simulink model "TorqueVect_HIL_CAN"  (R2022a)
settings: Solver=VariableStepAuto  StartTime=0.0  StopTime=300  RelTol=1e-3
PreLoadFcn:
  | run('Parameters\FSE_Parameters.m')
values from neighbouring files (symbols this model uses):
  Kd = 0;')    [open_carmaker_gui.m]
  Ki = 0    [open_carmaker_gui.m]
undefined symbols (not defined in the file or in its folder): BRegenEnabledButton, canChannel, CyalphaLookUp, efficiency, Fz_curve, Fz_scaling_long, gearR, izz, jw, kd, ki, Kp, kp, l_f, l_r, lambda, m, Mz_max, N, N_lat, N_long, P_max, pid_kd_lat, pid_kd_long, pid_ki_lat, pid_ki_long, pid_kp_lat, pid_kp_long, R_max, rw, steerR, T_i_max, TC_Decr_Gas, TC_Derivative, TC_Incr_Gas, TC_On, TC_Relay_Off, TC_Relay_On, tireCornerStiffness, Ts, TV_On, TV_Override, velocity_lookup, velocity_lookup_lat, y_ref, yrr_scaling
libraries: simulink x218, slpidlib x135, CarMaker4SL x73, TractionControlLibrary x13, canmsglib x11, canlib x10, TorqueVectoringLibrary x6, simulink_extras x4, PedalConversionLibrary x3, PowerControlLibrary x1
(part 19 of 26)

== system TorqueVect_HIL_CAN/CarMaker/IPG Vehicle/PowerTrain/PTControl Example/PTControl_PC_MFE/Subsystem/PowerControl/RegenError ==
  PTotal : Inport  Unit=W  PortDimensions=1
      settings: AttributesFormatString=%<Unit>
  FF_RC : Inport  Port=2
  PRegenLimit : Inport  Port=3  OutMin=0  OutMax=80000  Unit=W  PortDimensions=1
      settings: AttributesFormatString=[%<OutMin>, %<OutMax>] %<Unit>
  rThrottle : Inport  Port=4
  Product : Product
  Product6 : Product
  Saturation : Saturate  UpperLimit=0  LowerLimit=-250000
  Saturation7 : Saturate  UpperLimit=0  LowerLimit=-250000
      settings: AttributesFormatString=[%<LowerLimit>, %<UpperLimit>] W
  Subtract1 : Sum  Inputs=+-
  PRegenError : Outport  Unit=W  PortDimensions=1
      settings: AttributesFormatString=%<Unit>
  wires:
  Saturation/1 -> Subtract1/2
  PRegenLimit/1 -> Product/2
  rThrottle/1 -> Product/1
  Product/1 -> Saturation/1
  Subtract1/1 -> Saturation7/1
  PTotal/1 -> Product6/1
  Product6/1 -> Subtract1/1
  FF_RC/1 -> Product6/2
  Saturation7/1 -> PRegenError/1  "regen error"

== system TorqueVect_HIL_CAN/CarMaker/IPG Vehicle/PowerTrain/PTControl Example/PTControl_PC_MFE/Subsystem/PowerControl/ResetPID_PC ==
  rThrottlePedal : Inport
  BRegenEnabled : Inport  Port=2
  Derivative : Derivative
  Derivative1 : Derivative
  Detect Fall Negative : simulink/Logic and Bit Operations/Detect Fall Negative  vinit=0  OutDataTypeStr=boolean
      settings: SourceProductBaseCode=SL
  Detect Fall Negative1 : simulink/Logic and Bit Operations/Detect Fall Negative  vinit=0  OutDataTypeStr=boolean
      settings: SourceProductBaseCode=SL
  OR : Logic  Operator=OR  IconShape=distinctive  AllPortsSameDT=off  OutDataTypeStr=boolean
  ResetPID_PC : Outport
  wires:
  BRegenEnabled/1 -> Derivative/1
  Detect Fall Negative/1 -> OR/1  "regen_enable_or"
  Derivative1/1 -> Detect Fall Negative1/1
  rThrottlePedal/1 -> Derivative1/1
  Derivative/1 -> Detect Fall Negative/1
  Detect Fall Negative1/1 -> OR/2  "accel_pedal_falling_or"
  OR/1 -> ResetPID_PC/1

== system TorqueVect_HIL_CAN/CarMaker/IPG Vehicle/PowerTrain/PTControl Example/PTControl_PC_MFE/Subsystem/PowerControl/TotalPower ==
  MMotorFL : Inport  OutMin=-42  OutMax=42  Unit=N*m  PortDimensions=1
      settings: AttributesFormatString=[%<OutMin>, %<OutMax>] %<Unit>
  nMotorFL : Inport  Port=2  OutMin=-3000  OutMax=3000  Unit=rad/s  PortDimensions=1
      settings: AttributesFormatString=[%<OutMin>, %<OutMax>] %<Unit>
  MMotorFR : Inport  Port=3  OutMin=-42  OutMax=42  Unit=N*m  PortDimensions=1
      settings: AttributesFormatString=[%<OutMin>, %<OutMax>] %<Unit>
  nMotorFR : Inport  Port=4  OutMin=-3000  OutMax=3000  Unit=rad/s  PortDimensions=1
      settings: AttributesFormatString=[%<OutMin>, %<OutMax>] %<Unit>
  MMotorRL : Inport  Port=5  OutMin=-42  OutMax=42  Unit=N*m  PortDimensions=1
      settings: AttributesFormatString=[%<OutMin>, %<OutMax>] %<Unit>
  nMotorRL : Inport  Port=6  OutMin=-3000  OutMax=3000  Unit=rad/s  PortDimensions=1
      settings: AttributesFormatString=[%<OutMin>, %<OutMax>] %<Unit>
  MMotorRR : Inport  Port=7  OutMin=-42  OutMax=42  Unit=N*m  PortDimensions=1
      settings: AttributesFormatString=[%<OutMin>, %<OutMax>] %<Unit>
  nMotorRR : Inport  Port=8  OutMin=-3000  OutMax=3000  Unit=rad/s  PortDimensions=1
      settings: AttributesFormatString=[%<OutMin>, %<OutMax>] %<Unit>
  PMeasured : Inport  Port=9  OutMin=-250000  OutMax=250000  Unit=W  PortDimensions=1
      settings: AttributesFormatString=[%<OutMin>, %<OutMax>] %<Unit>
  BMeasuredEnable : Inport  Port=10  OutMin=0  OutMax=1  PortDimensions=1
      settings: AttributesFormatString=[%<OutMin> / %<OutMax>]
  Product{2,7..9} (4 alike) : Product
  Saturation{1,3..5} (4 alike) : Saturate  UpperLimit=250000  LowerLimit=0
  Sum1 : Sum  Inputs=++++
  Sum3 : Sum  Inputs=++++
  Switch : Switch  Threshold=1  SaturateOnIntegerOverflow=off  InputSameDT=off
  Switch3 : Switch  Threshold=1  SaturateOnIntegerOverflow=off  InputSameDT=off
  PPositiveTotal : Outport  OutMin=0  OutMax=250000  Unit=W  PortDimensions=1
      settings: AttributesFormatString=[%<OutMin>, %<OutMax>] %<Unit>
  PTotal : Outport  Port=2  OutMin=-250000  OutMax=250000  Unit=W  PortDimensions=1
      settings: AttributesFormatString=[%<OutMin>, %<OutMax>] %<Unit>
  wires:
  MMotorRR/1 -> Product9/2
  nMotorRR/1 -> Product9/1
  nMotorRL/1 -> Product8/2
  MMotorRL/1 -> Product8/1
  nMotorFR/1 -> Product7/2
  MMotorFR/1 -> Product7/1
  nMotorFL/1 -> Product2/2
  MMotorFL/1 -> Product2/1
  Product9/1 -> Saturation5/1, Sum1/4
  Product8/1 -> Saturation4/1, Sum1/3
  Product7/1 -> Saturation3/1, Sum1/2
  BMeasuredEnable/1 -> Switch/2, Switch3/2
  Switch3/1 -> PTotal/1
  PMeasured/1 -> Switch/1, Switch3/1
  Switch/1 -> PPositiveTotal/1
  Sum1/1 -> Switch3/3  "tot_powerrrr_RC"
  Saturation1/1 -> Sum3/1
  Saturation4/1 -> Sum3/3
  Product2/1 -> Saturation1/1, Sum1/1
  Saturation5/1 -> Sum3/4
  Sum3/1 -> Switch/3  "tot_powerrrr_PC"
  Saturation3/1 -> Sum3/2

== system TorqueVect_HIL_CAN/CarMaker/IPG Vehicle/PowerTrain/PTControl Example/PTControl_PC_MFE/Subsystem/PowerControl/WheelTorqueOut ==
  PReductionF : Inport
  PReductionR : Inport  Port=2
  nMotorFL : Inport  Port=3
  nMotorFR : Inport  Port=4
  nMotorRL : Inport  Port=5
  nMotorRR : Inport  Port=6
  Divide{1..4} (4 alike) : Product  Inputs=*/
  Gain : Gain  Gain=0.5
  Gain1 : Gain  Gain=0.5
  Saturation{1..4} (4 alike) : Saturate  UpperLimit=30000  LowerLimit=1
  MReductionMotorFL : Outport
  MReductionMotorFR : Outport  Port=2
  MReductionMotorRL : Outport  Port=3
  MReductionMotorRR : Outport  Port=4
  wires:
  Divide4/1 -> MReductionMotorRR/1
  Divide3/1 -> MReductionMotorRL/1
  Divide2/1 -> MReductionMotorFR/1
  Divide1/1 -> MReductionMotorFL/1
  Saturation4/1 -> Divide4/2
  Saturation3/1 -> Divide3/2
  nMotorRR/1 -> Saturation4/1
  nMotorRL/1 -> Saturation3/1
  Gain1/1 -> Divide3/1, Divide4/1
  Saturation2/1 -> Divide2/2
  Saturation1/1 -> Divide1/2
  nMotorFR/1 -> Saturation2/1
  nMotorFL/1 -> Saturation1/1
  Gain/1 -> Divide1/1, Divide2/1
  PReductionR/1 -> Gain1/1
  PReductionF/1 -> Gain/1

== system TorqueVect_HIL_CAN/CarMaker/IPG Vehicle/PowerTrain/PTControl Example/PTControl_PC_TC_MFE/New TC/TC R1/traction_controller ==
  max_torque : Inport
  dslip : Inport  Port=2
  enable_tc : Inport  Port=3
  Kp : Inport  Port=4
  Kd : Inport  Port=5
  Add : Sum  Inputs=+-
  Saturation Dynamic : simulink/Discontinuities/Saturation Dynamic  OutMin=[]  OutMax=[]  OutDataTypeStr=Inherit: Same as second input  OutDataType=fixdt(1, 16)  OutScaling=2^-10  DoSatur=off
  min_torque : Constant  Value=0
  traction_controller : Subsystem  TreatAsAtomicUnit=on
  delta_torque : Outport  VectorParamsAs1DForOutWhenUnconnected=off
  wires:
  Kd/1 -> traction_controller/4(Kd)
  enable_tc/1 -> traction_controller/2(enable_tc)
  Kp/1 -> traction_controller/3(Kp)
  traction_controller/1(delta_torque) -> Add/2
  dslip/1 -> traction_controller/1(dslip)
  Saturation Dynamic/1 -> delta_torque/1
  max_torque/1 -> Add/1, Saturation Dynamic/1
  min_torque/1 -> Saturation Dynamic/3
  Add/1 -> Saturation Dynamic/2

== system TorqueVect_HIL_CAN/CarMaker/IPG Vehicle/PowerTrain/PTControl Example/PTControl_PC_TC_MFE/New TC/TC R2/traction_controller ==
  max_torque : Inport
  dslip : Inport  Port=2
  enable_tc : Inport  Port=3
  Kp : Inport  Port=4
  Kd : Inport  Port=5
  Add : Sum  Inputs=+-
  Saturation Dynamic : simulink/Discontinuities/Saturation Dynamic  OutMin=[]  OutMax=[]  OutDataTypeStr=Inherit: Same as second input  OutDataType=fixdt(1, 16)  OutScaling=2^-10  DoSatur=off
  min_torque : Constant  Value=0
  traction_controller : Subsystem  TreatAsAtomicUnit=on
  delta_torque : Outport  VectorParamsAs1DForOutWhenUnconnected=off
  wires:
  Kd/1 -> traction_controller/4(Kd)
  enable_tc/1 -> traction_controller/2(enable_tc)
  Kp/1 -> traction_controller/3(Kp)
  traction_controller/1(delta_torque) -> Add/2
  dslip/1 -> traction_controller/1(dslip)
  Saturation Dynamic/1 -> delta_torque/1
  max_torque/1 -> Add/1, Saturation Dynamic/1
  min_torque/1 -> Saturation Dynamic/3
  Add/1 -> Saturation Dynamic/2

== system TorqueVect_HIL_CAN/CarMaker/IPG Vehicle/PowerTrain/PTControl Example/PTControl_PC_TC_MFE/New TC/TC R3/traction_controller ==
  max_torque : Inport
  dslip : Inport  Port=2
  enable_tc : Inport  Port=3
  Kp : Inport  Port=4
  Kd : Inport  Port=5
  Add : Sum  Inputs=+-
  Saturation Dynamic : simulink/Discontinuities/Saturation Dynamic  OutMin=[]  OutMax=[]  OutDataTypeStr=Inherit: Same as second input  OutDataType=fixdt(1, 16)  OutScaling=2^-10  DoSatur=off
  min_torque : Constant  Value=0
  traction_controller : Subsystem  TreatAsAtomicUnit=on
  delta_torque : Outport  VectorParamsAs1DForOutWhenUnconnected=off
  wires:
  Kd/1 -> traction_controller/4(Kd)
  enable_tc/1 -> traction_controller/2(enable_tc)
  Kp/1 -> traction_controller/3(Kp)
  traction_controller/1(delta_torque) -> Add/2
  dslip/1 -> traction_controller/1(dslip)
  Saturation Dynamic/1 -> delta_torque/1
  max_torque/1 -> Add/1, Saturation Dynamic/1
  min_torque/1 -> Saturation Dynamic/3
  Add/1 -> Saturation Dynamic/2

== system TorqueVect_HIL_CAN/CarMaker/IPG Vehicle/PowerTrain/PTControl Example/PTControl_PC_TC_MFE/New TC/TC R4/traction_controller ==
  max_torque : Inport
  dslip : Inport  Port=2
  enable_tc : Inport  Port=3
  Kp : Inport  Port=4
  Kd : Inport  Port=5
  Add : Sum  Inputs=+-
  Saturation Dynamic : simulink/Discontinuities/Saturation Dynamic  OutMin=[]  OutMax=[]  OutDataTypeStr=Inherit: Same as second input  OutDataType=fixdt(1, 16)  OutScaling=2^-10  DoSatur=off
  min_torque : Constant  Value=0
  traction_controller : Subsystem  TreatAsAtomicUnit=on
  delta_torque : Outport  VectorParamsAs1DForOutWhenUnconnected=off
  wires:
  Kd/1 -> traction_controller/4(Kd)
  enable_tc/1 -> traction_controller/2(enable_tc)
  Kp/1 -> traction_controller/3(Kp)
  traction_controller/1(delta_torque) -> Add/2
  dslip/1 -> traction_controller/1(dslip)
  Saturation Dynamic/1 -> delta_torque/1
  max_torque/1 -> Add/1, Saturation Dynamic/1
  min_torque/1 -> Saturation Dynamic/3
  Add/1 -> Saturation Dynamic/2

== system TorqueVect_HIL_CAN/CarMaker/IPG Vehicle/PowerTrain/PTControl Example/PTControl_TC_MFE/New TC/TC R1/traction_controller ==
  max_torque : Inport
  dslip : Inport  Port=2
  enable_tc : Inport  Port=3
  Kp : Inport  Port=4
  Kd : Inport  Port=5
  Add : Sum  Inputs=+-
  Saturation Dynamic : simulink/Discontinuities/Saturation Dynamic  OutMin=[]  OutMax=[]  OutDataTypeStr=Inherit: Same as second input  OutDataType=fixdt(1, 16)  OutScaling=2^-10  DoSatur=off
  min_torque : Constant  Value=0
  traction_controller : Subsystem  TreatAsAtomicUnit=on
  delta_torque : Outport  VectorParamsAs1DForOutWhenUnconnected=off
  wires:
  Kd/1 -> traction_controller/4(Kd)
  enable_tc/1 -> traction_controller/2(enable_tc)
  Kp/1 -> traction_controller/3(Kp)
  traction_controller/1(delta_torque) -> Add/2
  dslip/1 -> traction_controller/1(dslip)
  Saturation Dynamic/1 -> delta_torque/1
  max_torque/1 -> Add/1, Saturation Dynamic/1
  min_torque/1 -> Saturation Dynamic/3
  Add/1 -> Saturation Dynamic/2

== system TorqueVect_HIL_CAN/CarMaker/IPG Vehicle/PowerTrain/PTControl Example/PTControl_TC_MFE/New TC/TC R2/traction_controller ==
  max_torque : Inport
  dslip : Inport  Port=2
  enable_tc : Inport  Port=3
  Kp : Inport  Port=4
  Kd : Inport  Port=5
  Add : Sum  Inputs=+-
  Saturation Dynamic : simulink/Discontinuities/Saturation Dynamic  OutMin=[]  OutMax=[]  OutDataTypeStr=Inherit: Same as second input  OutDataType=fixdt(1, 16)  OutScaling=2^-10  DoSatur=off
  min_torque : Constant  Value=0
  traction_controller : Subsystem  TreatAsAtomicUnit=on
  delta_torque : Outport  VectorParamsAs1DForOutWhenUnconnected=off
  wires:
  Kd/1 -> traction_controller/4(Kd)
  enable_tc/1 -> traction_controller/2(enable_tc)
  Kp/1 -> traction_controller/3(Kp)
  traction_controller/1(delta_torque) -> Add/2
  dslip/1 -> traction_controller/1(dslip)
  Saturation Dynamic/1 -> delta_torque/1
  max_torque/1 -> Add/1, Saturation Dynamic/1
  min_torque/1 -> Saturation Dynamic/3
  Add/1 -> Saturation Dynamic/2

== system TorqueVect_HIL_CAN/CarMaker/IPG Vehicle/PowerTrain/PTControl Example/PTControl_TC_MFE/New TC/TC R3/traction_controller ==
  max_torque : Inport
  dslip : Inport  Port=2
  enable_tc : Inport  Port=3
  Kp : Inport  Port=4
  Kd : Inport  Port=5
  Add : Sum  Inputs=+-
  Saturation Dynamic : simulink/Discontinuities/Saturation Dynamic  OutMin=[]  OutMax=[]  OutDataTypeStr=Inherit: Same as second input  OutDataType=fixdt(1, 16)  OutScaling=2^-10  DoSatur=off
  min_torque : Constant  Value=0
  traction_controller : Subsystem  TreatAsAtomicUnit=on
  delta_torque : Outport  VectorParamsAs1DForOutWhenUnconnected=off
  wires:
  Kd/1 -> traction_controller/4(Kd)
  enable_tc/1 -> traction_controller/2(enable_tc)
  Kp/1 -> traction_controller/3(Kp)
  traction_controller/1(delta_torque) -> Add/2
  dslip/1 -> traction_controller/1(dslip)
  Saturation Dynamic/1 -> delta_torque/1
  max_torque/1 -> Add/1, Saturation Dynamic/1
  min_torque/1 -> Saturation Dynamic/3
  Add/1 -> Saturation Dynamic/2

== system TorqueVect_HIL_CAN/CarMaker/IPG Vehicle/PowerTrain/PTControl Example/PTControl_TC_MFE/New TC/TC R4/traction_controller ==
  max_torque : Inport
  dslip : Inport  Port=2
  enable_tc : Inport  Port=3
  Kp : Inport  Port=4
  Kd : Inport  Port=5
  Add : Sum  Inputs=+-
  Saturation Dynamic : simulink/Discontinuities/Saturation Dynamic  OutMin=[]  OutMax=[]  OutDataTypeStr=Inherit: Same as second input  OutDataType=fixdt(1, 16)  OutScaling=2^-10  DoSatur=off
  min_torque : Constant  Value=0
  traction_controller : Subsystem  TreatAsAtomicUnit=on
  delta_torque : Outport  VectorParamsAs1DForOutWhenUnconnected=off
  wires:
  Kd/1 -> traction_controller/4(Kd)
  enable_tc/1 -> traction_controller/2(enable_tc)
  Kp/1 -> traction_controller/3(Kp)
  traction_controller/1(delta_torque) -> Add/2
  dslip/1 -> traction_controller/1(dslip)
  Saturation Dynamic/1 -> delta_torque/1
  max_torque/1 -> Add/1, Saturation Dynamic/1
  min_torque/1 -> Saturation Dynamic/3
  Add/1 -> Saturation Dynamic/2

== system TorqueVect_HIL_CAN/CarMaker/IPG Vehicle/PowerTrain/PTControl Example/PTControl_TV_IPG/Torque Control 0/Electronic Gas Pedal FL/Traction Control FL ==
  VC.Gas : Inport
  E_Gas. : Inport  Port=2
  Car.LongSlip : Inport  Port=3
  Add : Sum
  Compare To Constant : simulink/Logic and Bit Operations/Compare To Constant  relop=>  const=TC_Derivative  OutDataTypeStr=uint8  ZeroCross=off
  Derivative : Derivative
  Fcn : Fcn  Expr=u >0.05
  Fcn1 : Fcn  Expr=u+TC_Incr_Gas
  Fcn2 : Fcn  Expr=u-TC_Decr_Gas
  From : From
      settings: CloseFcn=tagdialog Close
  Goto : Goto
  Multiport Switch : MultiPortSwitch  DataPortOrder=Zero-based contiguous  zeroidx=on  SaturateOnIntegerOverflow=off  InputSameDT=off
  Relational Operator : RelationalOperator  Operator=<=  InputSameDT=off
  Relay : Relay  OnSwitchValue=TC_Relay_On  OffSwitchValue=TC_Relay_Off
  S-R Flip-Flop : simulink_extras/Flip Flops/S-R Flip-Flop  initial_condition=0
  Saturation : Saturate  UpperLimit=1  LowerLimit=0
  Saturation1 : Saturate  UpperLimit=1  LowerLimit=0
  Switch : Switch  Criteria=u2 > Threshold  SaturateOnIntegerOverflow=off  InputSameDT=off
  Terminator : Terminator
  E_Gas : Outport  VectorParamsAs1DForOutWhenUnconnected=off
  wires:
  From/1 -> Switch/3
  Saturation/1 -> Multiport Switch/4
  Fcn2/1 -> Saturation/1
  Saturation1/1 -> Switch/1
  Fcn1/1 -> Saturation1/1
  Relational Operator/1 -> S-R Flip-Flop/2
  Fcn/1 -> S-R Flip-Flop/1
  Switch/1 -> Multiport Switch/2
  S-R Flip-Flop/1 -> Switch/2
  S-R Flip-Flop/2 -> Terminator/1
  E_Gas./1 -> Multiport Switch/3, Fcn2/1, Fcn1/1, Relational Operator/2
  VC.Gas/1 -> Goto/1, Relational Operator/1
  Multiport Switch/1 -> E_Gas/1
  Add/1 -> Multiport Switch/1
  Compare To Constant/1 -> Add/2
  Derivative/1 -> Compare To Constant/1
  Relay/1 -> Add/1
  Car.LongSlip/1 -> Fcn/1, Derivative/1, Relay/1

== system TorqueVect_HIL_CAN/CarMaker/IPG Vehicle/PowerTrain/PTControl Example/PTControl_TV_IPG/Torque Control 1/Electronic Gas Pedal FR/Traction Control FR ==
  VC.Gas : Inport
  E_Gas. : Inport  Port=2
  Car.LongSlip : Inport  Port=3
  Add : Sum
  Compare To Constant : simulink/Logic and Bit Operations/Compare To Constant  relop=>  const=TC_Derivative  OutDataTypeStr=uint8  ZeroCross=off
  Derivative : Derivative
  Fcn : Fcn  Expr=u >0.05
  Fcn1 : Fcn  Expr=u+TC_Incr_Gas
  Fcn2 : Fcn  Expr=u-TC_Decr_Gas
  From : From
      settings: CloseFcn=tagdialog Close
  Goto : Goto
  Multiport Switch : MultiPortSwitch  DataPortOrder=Zero-based contiguous  zeroidx=on  SaturateOnIntegerOverflow=off  InputSameDT=off
  Relational Operator : RelationalOperator  Operator=<=  InputSameDT=off
  Relay : Relay  OnSwitchValue=TC_Relay_On  OffSwitchValue=TC_Relay_Off
  S-R Flip-Flop : simulink_extras/Flip Flops/S-R Flip-Flop  initial_condition=0
  Saturation : Saturate  UpperLimit=1  LowerLimit=0
  Saturation1 : Saturate  UpperLimit=1  LowerLimit=0
  Switch : Switch  Criteria=u2 > Threshold  SaturateOnIntegerOverflow=off  InputSameDT=off
  Terminator : Terminator
  E_Gas : Outport  VectorParamsAs1DForOutWhenUnconnected=off
  wires:
  Car.LongSlip/1 -> Relay/1, Derivative/1, Fcn/1
  Relay/1 -> Add/1
  Derivative/1 -> Compare To Constant/1
  Compare To Constant/1 -> Add/2
  Add/1 -> Multiport Switch/1
  Multiport Switch/1 -> E_Gas/1
  VC.Gas/1 -> Relational Operator/1, Goto/1
  E_Gas./1 -> Relational Operator/2, Fcn1/1, Fcn2/1, Multiport Switch/3
  S-R Flip-Flop/2 -> Terminator/1
  S-R Flip-Flop/1 -> Switch/2
  Switch/1 -> Multiport Switch/2
  Fcn/1 -> S-R Flip-Flop/1
  Relational Operator/1 -> S-R Flip-Flop/2
  Fcn1/1 -> Saturation1/1
  Saturation1/1 -> Switch/1
  Fcn2/1 -> Saturation/1
  Saturation/1 -> Multiport Switch/4
  From/1 -> Switch/3

== system TorqueVect_HIL_CAN/CarMaker/IPG Vehicle/PowerTrain/PTControl Example/PTControl_TV_IPG/Torque Control 2/Electronic Gas Pedal RL/Traction Control RL ==
  VC.Gas : Inport
  E_Gas. : Inport  Port=2
  Car.LongSlip : Inport  Port=3
  Add : Sum
  Compare To Constant : simulink/Logic and Bit Operations/Compare To Constant  relop=>  const=TC_Derivative  OutDataTypeStr=uint8  ZeroCross=off
  Derivative : Derivative
  Fcn : Fcn  Expr=u >0.05
  Fcn1 : Fcn  Expr=u+TC_Incr_Gas
  Fcn2 : Fcn  Expr=u-TC_Decr_Gas
  From : From
      settings: CloseFcn=tagdialog Close
  Goto : Goto
  Multiport Switch : MultiPortSwitch  DataPortOrder=Zero-based contiguous  zeroidx=on  SaturateOnIntegerOverflow=off  InputSameDT=off
  Relational Operator : RelationalOperator  Operator=<=  InputSameDT=off
  Relay : Relay  OnSwitchValue=TC_Relay_On  OffSwitchValue=TC_Relay_Off
  S-R Flip-Flop : simulink_extras/Flip Flops/S-R Flip-Flop  initial_condition=0
  Saturation : Saturate  UpperLimit=1  LowerLimit=0
  Saturation1 : Saturate  UpperLimit=1  LowerLimit=0
  Switch : Switch  Criteria=u2 > Threshold  SaturateOnIntegerOverflow=off  InputSameDT=off
  Terminator : Terminator
  E_Gas : Outport  VectorParamsAs1DForOutWhenUnconnected=off
  wires:
  Car.LongSlip/1 -> Relay/1, Derivative/1, Fcn/1
  Relay/1 -> Add/1
  Derivative/1 -> Compare To Constant/1
  Compare To Constant/1 -> Add/2
  Add/1 -> Multiport Switch/1
  Multiport Switch/1 -> E_Gas/1
  VC.Gas/1 -> Relational Operator/1, Goto/1
  E_Gas./1 -> Relational Operator/2, Fcn1/1, Fcn2/1, Multiport Switch/3
  S-R Flip-Flop/2 -> Terminator/1
  S-R Flip-Flop/1 -> Switch/2
  Switch/1 -> Multiport Switch/2
  Fcn/1 -> S-R Flip-Flop/1
  Relational Operator/1 -> S-R Flip-Flop/2
  Fcn1/1 -> Saturation1/1
  Saturation1/1 -> Switch/1
  Fcn2/1 -> Saturation/1
  Saturation/1 -> Multiport Switch/4
  From/1 -> Switch/3

== system TorqueVect_HIL_CAN/CarMaker/IPG Vehicle/PowerTrain/PTControl Example/PTControl_TV_IPG/Torque Control 3/Electronic Gas Pedal RR/Traction Control RR ==
  VC.Gas : Inport
  E_Gas. : Inport  Port=2
  Car.LongSlip : Inport  Port=3
  Add : Sum
  Compare To Constant : simulink/Logic and Bit Operations/Compare To Constant  relop=>  const=TC_Derivative  OutDataTypeStr=uint8  ZeroCross=off
  Derivative : Derivative
  Fcn : Fcn  Expr=u >0.05
  Fcn1 : Fcn  Expr=u+TC_Incr_Gas
  Fcn2 : Fcn  Expr=u-TC_Decr_Gas
  From : From
      settings: CloseFcn=tagdialog Close
  Goto : Goto
  Multiport Switch : MultiPortSwitch  DataPortOrder=Zero-based contiguous  zeroidx=on  SaturateOnIntegerOverflow=off  InputSameDT=off
  Relational Operator : RelationalOperator  Operator=<=  InputSameDT=off
  Relay : Relay  OnSwitchValue=TC_Relay_On  OffSwitchValue=TC_Relay_Off
  S-R Flip-Flop : simulink_extras/Flip Flops/S-R Flip-Flop  initial_condition=0
  Saturation : Saturate  UpperLimit=1  LowerLimit=0
  Saturation1 : Saturate  UpperLimit=1  LowerLimit=0
  Switch : Switch  Criteria=u2 > Threshold  SaturateOnIntegerOverflow=off  InputSameDT=off
  Terminator : Terminator
  E_Gas : Outport  VectorParamsAs1DForOutWhenUnconnected=off
  wires:
  From/1 -> Switch/3
  Saturation/1 -> Multiport Switch/4
  Fcn2/1 -> Saturation/1
  Saturation1/1 -> Switch/1
  Fcn1/1 -> Saturation1/1
  Relational Operator/1 -> S-R Flip-Flop/2
  Fcn/1 -> S-R Flip-Flop/1
  Switch/1 -> Multiport Switch/2
  S-R Flip-Flop/1 -> Switch/2
  S-R Flip-Flop/2 -> Terminator/1
  E_Gas./1 -> Multiport Switch/3, Fcn2/1, Fcn1/1, Relational Operator/2
  VC.Gas/1 -> Goto/1, Relational Operator/1
  Multiport Switch/1 -> E_Gas/1
  Add/1 -> Multiport Switch/1
  Compare To Constant/1 -> Add/2
  Derivative/1 -> Compare To Constant/1
  Relay/1 -> Add/1
  Car.LongSlip/1 -> Fcn/1, Derivative/1, Relay/1

== system TorqueVect_HIL_CAN/CarMaker/IPG Vehicle/PowerTrain/PTControl Example/PTControl_TV_MFE1/New TC/TC R1/traction_controller ==
  max_torque : Inport
  dslip : Inport  Port=2
  enable_tc : Inport  Port=3
  Kp : Inport  Port=4
  Kd : Inport  Port=5
  Add : Sum  Inputs=+-
  Saturation Dynamic : simulink/Discontinuities/Saturation Dynamic  OutMin=[]  OutMax=[]  OutDataTypeStr=Inherit: Same as second input  OutDataType=fixdt(1, 16)  OutScaling=2^-10  DoSatur=off
  min_torque : Constant  Value=0
  traction_controller : Subsystem  TreatAsAtomicUnit=on
  delta_torque : Outport  VectorParamsAs1DForOutWhenUnconnected=off
  wires:
  Kd/1 -> traction_controller/4(Kd)
  enable_tc/1 -> traction_controller/2(enable_tc)
  Kp/1 -> traction_controller/3(Kp)
  traction_controller/1(delta_torque) -> Add/2
  dslip/1 -> traction_controller/1(dslip)
  Saturation Dynamic/1 -> delta_torque/1
  max_torque/1 -> Add/1, Saturation Dynamic/1
  min_torque/1 -> Saturation Dynamic/3
  Add/1 -> Saturation Dynamic/2

== system TorqueVect_HIL_CAN/CarMaker/IPG Vehicle/PowerTrain/PTControl Example/PTControl_TV_MFE1/New TC/TC R2/traction_controller ==
  max_torque : Inport
  dslip : Inport  Port=2
  enable_tc : Inport  Port=3
  Kp : Inport  Port=4
  Kd : Inport  Port=5
  Add : Sum  Inputs=+-
  Saturation Dynamic : simulink/Discontinuities/Saturation Dynamic  OutMin=[]  OutMax=[]  OutDataTypeStr=Inherit: Same as second input  OutDataType=fixdt(1, 16)  OutScaling=2^-10  DoSatur=off
  min_torque : Constant  Value=0
  traction_controller : Subsystem  TreatAsAtomicUnit=on
  delta_torque : Outport  VectorParamsAs1DForOutWhenUnconnected=off
  wires:
  Kd/1 -> traction_controller/4(Kd)
  enable_tc/1 -> traction_controller/2(enable_tc)
  Kp/1 -> traction_controller/3(Kp)
  traction_controller/1(delta_torque) -> Add/2
  dslip/1 -> traction_controller/1(dslip)
  Saturation Dynamic/1 -> delta_torque/1
  max_torque/1 -> Add/1, Saturation Dynamic/1
  min_torque/1 -> Saturation Dynamic/3
  Add/1 -> Saturation Dynamic/2

== system TorqueVect_HIL_CAN/CarMaker/IPG Vehicle/PowerTrain/PTControl Example/PTControl_TV_MFE1/New TC/TC R3/traction_controller ==
  max_torque : Inport
  dslip : Inport  Port=2
  enable_tc : Inport  Port=3
  Kp : Inport  Port=4
  Kd : Inport  Port=5
  Add : Sum  Inputs=+-
  Saturation Dynamic : simulink/Discontinuities/Saturation Dynamic  OutMin=[]  OutMax=[]  OutDataTypeStr=Inherit: Same as second input  OutDataType=fixdt(1, 16)  OutScaling=2^-10  DoSatur=off
  min_torque : Constant  Value=0
  traction_controller : Subsystem  TreatAsAtomicUnit=on
  delta_torque : Outport  VectorParamsAs1DForOutWhenUnconnected=off
  wires:
  Kd/1 -> traction_controller/4(Kd)
  enable_tc/1 -> traction_controller/2(enable_tc)
  Kp/1 -> traction_controller/3(Kp)
  traction_controller/1(delta_torque) -> Add/2
  dslip/1 -> traction_controller/1(dslip)
  Saturation Dynamic/1 -> delta_torque/1
  max_torque/1 -> Add/1, Saturation Dynamic/1
  min_torque/1 -> Saturation Dynamic/3
  Add/1 -> Saturation Dynamic/2

== system TorqueVect_HIL_CAN/CarMaker/IPG Vehicle/PowerTrain/PTControl Example/PTControl_TV_MFE1/New TC/TC R4/traction_controller ==
  max_torque : Inport
  dslip : Inport  Port=2
  enable_tc : Inport  Port=3
  Kp : Inport  Port=4
  Kd : Inport  Port=5
  Add : Sum  Inputs=+-
  Saturation Dynamic : simulink/Discontinuities/Saturation Dynamic  OutMin=[]  OutMax=[]  OutDataTypeStr=Inherit: Same as second input  OutDataType=fixdt(1, 16)  OutScaling=2^-10  DoSatur=off
  min_torque : Constant  Value=0
  traction_controller : Subsystem  TreatAsAtomicUnit=on
  delta_torque : Outport  VectorParamsAs1DForOutWhenUnconnected=off
  wires:
  Kd/1 -> traction_controller/4(Kd)
  enable_tc/1 -> traction_controller/2(enable_tc)
  Kp/1 -> traction_controller/3(Kp)
  traction_controller/1(delta_torque) -> Add/2
  dslip/1 -> traction_controller/1(dslip)
  Saturation Dynamic/1 -> delta_torque/1
  max_torque/1 -> Add/1, Saturation Dynamic/1
  min_torque/1 -> Saturation Dynamic/3
  Add/1 -> Saturation Dynamic/2

== system TorqueVect_HIL_CAN/CarMaker/IPG Vehicle/PowerTrain/PTControl Example/PTControl_TV_MFE1/Subsystem/TorqueVectoringAlgorithm/If Action Subsystem ==
  NTorqueWheel : Inport
  NTorqueDelta : Inport  Port=2
  Action Port : ActionPort
  Add : Sum  Inputs=+-
  Add1 : Sum
  NTorqueLeftOut : Outport
  NTorqueRightOut : Outport  Port=2
  wires:
  NTorqueDelta/1 -> Add/2, Add1/2
  NTorqueWheel/1 -> Add/1, Add1/1
  Add1/1 -> NTorqueRightOut/1
  Add/1 -> NTorqueLeftOut/1

== system TorqueVect_HIL_CAN/CarMaker/IPG Vehicle/PowerTrain/PTControl Example/PTControl_TV_MFE1/Subsystem/TorqueVectoringAlgorithm/If Action Subsystem1 ==
  NTorqueWheel : Inport
  NTorqueWheel1 : Inport  Port=2
  Action Port : ActionPort
  NTorqueLeftOut : Outport
  NTorqueRightOut : Outport  Port=2
  wires:
  NTorqueWheel/1 -> NTorqueLeftOut/1
  NTorqueWheel1/1 -> NTorqueRightOut/1

== system TorqueVect_HIL_CAN/CarMaker/IPG Vehicle/PowerTrain/PTControl Example/PTControl_TV_MFE1/Subsystem/TorqueVectoringAlgorithm1/If Action Subsystem ==
  NTorqueWheel : Inport
  NTorqueDelta : Inport  Port=2
  Action Port : ActionPort
  Add : Sum  Inputs=+-
  Add1 : Sum
  NTorqueLeftOut : Outport
  NTorqueRightOut : Outport  Port=2
  wires:
  NTorqueDelta/1 -> Add/2, Add1/2
  NTorqueWheel/1 -> Add/1, Add1/1
  Add1/1 -> NTorqueRightOut/1
  Add/1 -> NTorqueLeftOut/1

== system TorqueVect_HIL_CAN/CarMaker/IPG Vehicle/PowerTrain/PTControl Example/PTControl_TV_MFE1/Subsystem/TorqueVectoringAlgorithm1/If Action Subsystem1 ==
  NTorqueWheel : Inport
  NTorqueWheel1 : Inport  Port=2
  Action Port : ActionPort
  NTorqueLeftOut : Outport
  NTorqueRightOut : Outport  Port=2
  wires:
  NTorqueWheel/1 -> NTorqueLeftOut/1
  NTorqueWheel1/1 -> NTorqueRightOut/1

== system TorqueVect_HIL_CAN/CarMaker/IPG Vehicle/PowerTrain/PTControl Example/PTControl_TV_MFE2/New TC/TC R1/traction_controller ==
  max_torque : Inport
  dslip : Inport  Port=2
  enable_tc : Inport  Port=3
  Kp : Inport  Port=4
  Kd : Inport  Port=5
  Add : Sum  Inputs=+-
  Saturation Dynamic : simulink/Discontinuities/Saturation Dynamic  OutMin=[]  OutMax=[]  OutDataTypeStr=Inherit: Same as second input  OutDataType=fixdt(1, 16)  OutScaling=2^-10  DoSatur=off
  min_torque : Constant  Value=0
  traction_controller : Subsystem  TreatAsAtomicUnit=on
  delta_torque : Outport  VectorParamsAs1DForOutWhenUnconnected=off
  wires:
  Kd/1 -> traction_controller/4(Kd)
  enable_tc/1 -> traction_controller/2(enable_tc)
  Kp/1 -> traction_controller/3(Kp)
  traction_controller/1(delta_torque) -> Add/2
  dslip/1 -> traction_controller/1(dslip)
  Saturation Dynamic/1 -> delta_torque/1
  max_torque/1 -> Add/1, Saturation Dynamic/1
  min_torque/1 -> Saturation Dynamic/3
  Add/1 -> Saturation Dynamic/2

== system TorqueVect_HIL_CAN/CarMaker/IPG Vehicle/PowerTrain/PTControl Example/PTControl_TV_MFE2/New TC/TC R2/traction_controller ==
  max_torque : Inport
  dslip : Inport  Port=2
  enable_tc : Inport  Port=3
  Kp : Inport  Port=4
  Kd : Inport  Port=5
  Add : Sum  Inputs=+-
  Saturation Dynamic : simulink/Discontinuities/Saturation Dynamic  OutMin=[]  OutMax=[]  OutDataTypeStr=Inherit: Same as second input  OutDataType=fixdt(1, 16)  OutScaling=2^-10  DoSatur=off
  min_torque : Constant  Value=0
  traction_controller : Subsystem  TreatAsAtomicUnit=on
  delta_torque : Outport  VectorParamsAs1DForOutWhenUnconnected=off
  wires:
  Kd/1 -> traction_controller/4(Kd)
  enable_tc/1 -> traction_controller/2(enable_tc)
  Kp/1 -> traction_controller/3(Kp)
  traction_controller/1(delta_torque) -> Add/2
  dslip/1 -> traction_controller/1(dslip)
  Saturation Dynamic/1 -> delta_torque/1
  max_torque/1 -> Add/1, Saturation Dynamic/1
  min_torque/1 -> Saturation Dynamic/3
  Add/1 -> Saturation Dynamic/2

== system TorqueVect_HIL_CAN/CarMaker/IPG Vehicle/PowerTrain/PTControl Example/PTControl_TV_MFE2/New TC/TC R3/traction_controller ==
  max_torque : Inport
  dslip : Inport  Port=2
  enable_tc : Inport  Port=3
  Kp : Inport  Port=4
  Kd : Inport  Port=5
  Add : Sum  Inputs=+-
  Saturation Dynamic : simulink/Discontinuities/Saturation Dynamic  OutMin=[]  OutMax=[]  OutDataTypeStr=Inherit: Same as second input  OutDataType=fixdt(1, 16)  OutScaling=2^-10  DoSatur=off
  min_torque : Constant  Value=0
  traction_controller : Subsystem  TreatAsAtomicUnit=on
  delta_torque : Outport  VectorParamsAs1DForOutWhenUnconnected=off
  wires:
  Kd/1 -> traction_controller/4(Kd)
  enable_tc/1 -> traction_controller/2(enable_tc)
  Kp/1 -> traction_controller/3(Kp)
  traction_controller/1(delta_torque) -> Add/2
  dslip/1 -> traction_controller/1(dslip)
  Saturation Dynamic/1 -> delta_torque/1
  max_torque/1 -> Add/1, Saturation Dynamic/1
  min_torque/1 -> Saturation Dynamic/3
  Add/1 -> Saturation Dynamic/2

== system TorqueVect_HIL_CAN/CarMaker/IPG Vehicle/PowerTrain/PTControl Example/PTControl_TV_MFE2/New TC/TC R4/traction_controller ==
  max_torque : Inport
  dslip : Inport  Port=2
  enable_tc : Inport  Port=3
  Kp : Inport  Port=4
  Kd : Inport  Port=5
  Add : Sum  Inputs=+-
  Saturation Dynamic : simulink/Discontinuities/Saturation Dynamic  OutMin=[]  OutMax=[]  OutDataTypeStr=Inherit: Same as second input  OutDataType=fixdt(1, 16)  OutScaling=2^-10  DoSatur=off
  min_torque : Constant  Value=0
  traction_controller : Subsystem  TreatAsAtomicUnit=on
  delta_torque : Outport  VectorParamsAs1DForOutWhenUnconnected=off
  wires:
  Kd/1 -> traction_controller/4(Kd)
  enable_tc/1 -> traction_controller/2(enable_tc)
  Kp/1 -> traction_controller/3(Kp)
  traction_controller/1(delta_torque) -> Add/2
  dslip/1 -> traction_controller/1(dslip)
  Saturation Dynamic/1 -> delta_torque/1
  max_torque/1 -> Add/1, Saturation Dynamic/1
  min_torque/1 -> Saturation Dynamic/3
  Add/1 -> Saturation Dynamic/2

== system TorqueVect_HIL_CAN/CarMaker/IPG Vehicle/PowerTrain/PTControl Example/PTControl_TV_MFE2/Subsystem/TorqueVectoringAlgorithm/If Action Subsystem ==
  NTorqueWheel : Inport
  NTorqueDelta : Inport  Port=2
  Action Port : ActionPort
  Add : Sum  Inputs=+-
  Add1 : Sum
  NTorqueLeftOut : Outport
  NTorqueRightOut : Outport  Port=2
  wires:
  NTorqueDelta/1 -> Add/2, Add1/2
  NTorqueWheel/1 -> Add/1, Add1/1
  Add1/1 -> NTorqueRightOut/1
  Add/1 -> NTorqueLeftOut/1

== system TorqueVect_HIL_CAN/CarMaker/IPG Vehicle/PowerTrain/PTControl Example/PTControl_TV_MFE2/Subsystem/TorqueVectoringAlgorithm/If Action Subsystem1 ==
  NTorqueWheel : Inport
  NTorqueWheel1 : Inport  Port=2
  Action Port : ActionPort
  NTorqueLeftOut : Outport
  NTorqueRightOut : Outport  Port=2
  wires:
  NTorqueWheel/1 -> NTorqueLeftOut/1
  NTorqueWheel1/1 -> NTorqueRightOut/1

== system TorqueVect_HIL_CAN/CarMaker/IPG Vehicle/PowerTrain/PTControl Example/PTControl_TV_MFE2/Subsystem/TorqueVectoringAlgorithm1/If Action Subsystem ==
  NTorqueWheel : Inport
  NTorqueDelta : Inport  Port=2
  Action Port : ActionPort
  Add : Sum  Inputs=+-
  Add1 : Sum
  NTorqueLeftOut : Outport
  NTorqueRightOut : Outport  Port=2
  wires:
  NTorqueDelta/1 -> Add/2, Add1/2
  NTorqueWheel/1 -> Add/1, Add1/1
  Add1/1 -> NTorqueRightOut/1
  Add/1 -> NTorqueLeftOut/1

== system TorqueVect_HIL_CAN/CarMaker/IPG Vehicle/PowerTrain/PTControl Example/PTControl_TV_MFE2/Subsystem/TorqueVectoringAlgorithm1/If Action Subsystem1 ==
  NTorqueWheel : Inport
  NTorqueWheel1 : Inport  Port=2
  Action Port : ActionPort
  NTorqueLeftOut : Outport
  NTorqueRightOut : Outport  Port=2
  wires:
  NTorqueWheel/1 -> NTorqueLeftOut/1
  NTorqueWheel1/1 -> NTorqueRightOut/1

== system TorqueVect_HIL_CAN/CarMaker/IPG Vehicle/PowerTrain/PTControl Example/PTControl_TV_MFE25/Full Control Loop/TC 1/Subsystem ==
  velocity : Inport
  pid_kp : Inport  Port=2
  velocity lookup : Inport  Port=3
  pid_ki : Inport  Port=4
  pid_kd : Inport  Port=5
  kd : Lookup_n-D  NumberOfTableDimensions=1  BreakpointsForDimension1Source=Input port  BreakpointsForDimension1=[-5:5]  TableSource=Input port  Table=tanh([-5:5])  InternalRulePriority=Speed  RndMeth=Simplest
      settings: InputPortMap=u0,p221,p5
  ki : Lookup_n-D  NumberOfTableDimensions=1  BreakpointsForDimension1Source=Input port  BreakpointsForDimension1=[-5:5]  TableSource=Input port  Table=tanh([-5:5])  InternalRulePriority=Speed  RndMeth=Simplest
      settings: InputPortMap=u0,p221,p5
  kp : Lookup_n-D  NumberOfTableDimensions=1  BreakpointsForDimension1Source=Input port  BreakpointsForDimension1=[-5:5]  TableSource=Input port  Table=tanh([-5:5])  InternalRulePriority=Speed  RndMeth=Simplest
      settings: InputPortMap=u0,p221,p5
  Out1 : Outport
  Out2 : Outport  Port=2
  Out3 : Outport  Port=3
  wires:
  pid_kd/1 -> kd/2
  pid_ki/1 -> ki/2
  pid_kp/1 -> kp/2
  velocity lookup/1 -> kp/3, ki/3, kd/3
  ki/1 -> Out2/1
  kd/1 -> Out3/1
  velocity/1 -> ki/1, kd/1, kp/1
  kp/1 -> Out1/1

== system TorqueVect_HIL_CAN/CarMaker/IPG Vehicle/PowerTrain/PTControl Example/PTControl_TV_MFE25/Full Control Loop/TC 2/Subsystem ==
  velocity : Inport
  pid_kp : Inport  Port=2
  velocity lookup : Inport  Port=3
  pid_ki : Inport  Port=4
  pid_kd : Inport  Port=5
  kd : Lookup_n-D  NumberOfTableDimensions=1  BreakpointsForDimension1Source=Input port  BreakpointsForDimension1=[-5:5]  TableSource=Input port  Table=tanh([-5:5])  InternalRulePriority=Speed  RndMeth=Simplest
      settings: InputPortMap=u0,p221,p5
  ki : Lookup_n-D  NumberOfTableDimensions=1  BreakpointsForDimension1Source=Input port  BreakpointsForDimension1=[-5:5]  TableSource=Input port  Table=tanh([-5:5])  InternalRulePriority=Speed  RndMeth=Simplest
      settings: InputPortMap=u0,p221,p5
  kp : Lookup_n-D  NumberOfTableDimensions=1  BreakpointsForDimension1Source=Input port  BreakpointsForDimension1=[-5:5]  TableSource=Input port  Table=tanh([-5:5])  InternalRulePriority=Speed  RndMeth=Simplest
      settings: InputPortMap=u0,p221,p5
  Out1 : Outport
  Out2 : Outport  Port=2
  Out3 : Outport  Port=3
  wires:
  pid_kd/1 -> kd/2
  pid_ki/1 -> ki/2
  pid_kp/1 -> kp/2
  velocity lookup/1 -> kp/3, ki/3, kd/3
  ki/1 -> Out2/1
  kd/1 -> Out3/1
  velocity/1 -> ki/1, kd/1, kp/1
  kp/1 -> Out1/1

== system TorqueVect_HIL_CAN/CarMaker/IPG Vehicle/PowerTrain/PTControl Example/PTControl_TV_MFE25/Full Control Loop/TC 3/Subsystem ==
  velocity : Inport
  pid_kp : Inport  Port=2
  velocity lookup : Inport  Port=3
  pid_ki : Inport  Port=4
  pid_kd : Inport  Port=5
  kd : Lookup_n-D  NumberOfTableDimensions=1  BreakpointsForDimension1Source=Input port  BreakpointsForDimension1=[-5:5]  TableSource=Input port  Table=tanh([-5:5])  InternalRulePriority=Speed  RndMeth=Simplest
      settings: InputPortMap=u0,p221,p5
  ki : Lookup_n-D  NumberOfTableDimensions=1  BreakpointsForDimension1Source=Input port  BreakpointsForDimension1=[-5:5]  TableSource=Input port  Table=tanh([-5:5])  InternalRulePriority=Speed  RndMeth=Simplest
      settings: InputPortMap=u0,p221,p5
  kp : Lookup_n-D  NumberOfTableDimensions=1  BreakpointsForDimension1Source=Input port  BreakpointsForDimension1=[-5:5]  TableSource=Input port  Table=tanh([-5:5])  InternalRulePriority=Speed  RndMeth=Simplest
      settings: InputPortMap=u0,p221,p5
  Out1 : Outport
  Out2 : Outport  Port=2
  Out3 : Outport  Port=3
  wires:
  pid_kd/1 -> kd/2
  pid_ki/1 -> ki/2
  pid_kp/1 -> kp/2
  velocity lookup/1 -> kp/3, ki/3, kd/3
  ki/1 -> Out2/1
  kd/1 -> Out3/1
  velocity/1 -> ki/1, kd/1, kp/1
  kp/1 -> Out1/1

== system TorqueVect_HIL_CAN/CarMaker/IPG Vehicle/PowerTrain/PTControl Example/PTControl_TV_MFE25/Full Control Loop/TC 4/Subsystem ==
  velocity : Inport
  pid_kp : Inport  Port=2
  velocity lookup : Inport  Port=3
  pid_ki : Inport  Port=4
  pid_kd : Inport  Port=5
  kd : Lookup_n-D  NumberOfTableDimensions=1  BreakpointsForDimension1Source=Input port  BreakpointsForDimension1=[-5:5]  TableSource=Input port  Table=tanh([-5:5])  InternalRulePriority=Speed  RndMeth=Simplest
      settings: InputPortMap=u0,p221,p5
  ki : Lookup_n-D  NumberOfTableDimensions=1  BreakpointsForDimension1Source=Input port  BreakpointsForDimension1=[-5:5]  TableSource=Input port  Table=tanh([-5:5])  InternalRulePriority=Speed  RndMeth=Simplest
      settings: InputPortMap=u0,p221,p5
  kp : Lookup_n-D  NumberOfTableDimensions=1  BreakpointsForDimension1Source=Input port  BreakpointsForDimension1=[-5:5]  TableSource=Input port  Table=tanh([-5:5])  InternalRulePriority=Speed  RndMeth=Simplest
      settings: InputPortMap=u0,p221,p5
  Out1 : Outport
  Out2 : Outport  Port=2
  Out3 : Outport  Port=3
  wires:
  pid_kd/1 -> kd/2
  pid_ki/1 -> ki/2
  pid_kp/1 -> kp/2
  velocity lookup/1 -> kp/3, ki/3, kd/3
  ki/1 -> Out2/1
  kd/1 -> Out3/1
  velocity/1 -> ki/1, kd/1, kp/1
  kp/1 -> Out1/1

== system TorqueVect_HIL_CAN/CarMaker/IPG Vehicle/PowerTrain/PTControl Example/PTControl_TV_MFE25/New TC/TC R1/traction_controller ==
  max_torque : Inport
  dslip : Inport  Port=2
  enable_tc : Inport  Port=3
  Kp : Inport  Port=4
  Kd : Inport  Port=5
  Add : Sum  Inputs=+-
  Saturation Dynamic : simulink/Discontinuities/Saturation Dynamic  OutMin=[]  OutMax=[]  OutDataTypeStr=Inherit: Same as second input  OutDataType=fixdt(1, 16)  OutScaling=2^-10  DoSatur=off
  min_torque : Constant  Value=0
  traction_controller : Subsystem  TreatAsAtomicUnit=on
  delta_torque : Outport  VectorParamsAs1DForOutWhenUnconnected=off
  wires:
  Kd/1 -> traction_controller/4(Kd)
  enable_tc/1 -> traction_controller/2(enable_tc)
  Kp/1 -> traction_controller/3(Kp)
  traction_controller/1(delta_torque) -> Add/2
  dslip/1 -> traction_controller/1(dslip)
  Saturation Dynamic/1 -> delta_torque/1
  max_torque/1 -> Add/1, Saturation Dynamic/1
  min_torque/1 -> Saturation Dynamic/3
  Add/1 -> Saturation Dynamic/2

== system TorqueVect_HIL_CAN/CarMaker/IPG Vehicle/PowerTrain/PTControl Example/PTControl_TV_MFE25/New TC/TC R2/traction_controller ==
  max_torque : Inport
  dslip : Inport  Port=2
  enable_tc : Inport  Port=3
  Kp : Inport  Port=4
  Kd : Inport  Port=5
  Add : Sum  Inputs=+-
  Saturation Dynamic : simulink/Discontinuities/Saturation Dynamic  OutMin=[]  OutMax=[]  OutDataTypeStr=Inherit: Same as second input  OutDataType=fixdt(1, 16)  OutScaling=2^-10  DoSatur=off
  min_torque : Constant  Value=0
  traction_controller : Subsystem  TreatAsAtomicUnit=on
  delta_torque : Outport  VectorParamsAs1DForOutWhenUnconnected=off
  wires:
  Kd/1 -> traction_controller/4(Kd)
  enable_tc/1 -> traction_controller/2(enable_tc)
  Kp/1 -> traction_controller/3(Kp)
  traction_controller/1(delta_torque) -> Add/2
  dslip/1 -> traction_controller/1(dslip)
  Saturation Dynamic/1 -> delta_torque/1
  max_torque/1 -> Add/1, Saturation Dynamic/1
  min_torque/1 -> Saturation Dynamic/3
  Add/1 -> Saturation Dynamic/2

== system TorqueVect_HIL_CAN/CarMaker/IPG Vehicle/PowerTrain/PTControl Example/PTControl_TV_MFE25/New TC/TC R3/traction_controller ==
  max_torque : Inport
  dslip : Inport  Port=2
  enable_tc : Inport  Port=3
  Kp : Inport  Port=4
  Kd : Inport  Port=5
  Add : Sum  Inputs=+-
  Saturation Dynamic : simulink/Discontinuities/Saturation Dynamic  OutMin=[]  OutMax=[]  OutDataTypeStr=Inherit: Same as second input  OutDataType=fixdt(1, 16)  OutScaling=2^-10  DoSatur=off
  min_torque : Constant  Value=0
  traction_controller : Subsystem  TreatAsAtomicUnit=on
  delta_torque : Outport  VectorParamsAs1DForOutWhenUnconnected=off
  wires:
  Kd/1 -> traction_controller/4(Kd)
  enable_tc/1 -> traction_controller/2(enable_tc)
  Kp/1 -> traction_controller/3(Kp)
  traction_controller/1(delta_torque) -> Add/2
  dslip/1 -> traction_controller/1(dslip)
  Saturation Dynamic/1 -> delta_torque/1
  max_torque/1 -> Add/1, Saturation Dynamic/1
  min_torque/1 -> Saturation Dynamic/3
  Add/1 -> Saturation Dynamic/2

== system TorqueVect_HIL_CAN/CarMaker/IPG Vehicle/PowerTrain/PTControl Example/PTControl_TV_MFE25/New TC/TC R4/traction_controller ==
  max_torque : Inport
  dslip : Inport  Port=2
  enable_tc : Inport  Port=3
  Kp : Inport  Port=4
  Kd : Inport  Port=5
  Add : Sum  Inputs=+-
  Saturation Dynamic : simulink/Discontinuities/Saturation Dynamic  OutMin=[]  OutMax=[]  OutDataTypeStr=Inherit: Same as second input  OutDataType=fixdt(1, 16)  OutScaling=2^-10  DoSatur=off
  min_torque : Constant  Value=0
  traction_controller : Subsystem  TreatAsAtomicUnit=on
  delta_torque : Outport  VectorParamsAs1DForOutWhenUnconnected=off
  wires:
  Kd/1 -> traction_controller/4(Kd)
  enable_tc/1 -> traction_controller/2(enable_tc)
  Kp/1 -> traction_controller/3(Kp)
  traction_controller/1(delta_torque) -> Add/2
  dslip/1 -> traction_controller/1(dslip)
  Saturation Dynamic/1 -> delta_torque/1
  max_torque/1 -> Add/1, Saturation Dynamic/1
  min_torque/1 -> Saturation Dynamic/3
  Add/1 -> Saturation Dynamic/2

== system TorqueVect_HIL_CAN/CarMaker/IPG Vehicle/PowerTrain/PTControl Example/PTControl_TV_MFE25_2022a1/New TC/TC R1/traction_controller ==
  max_torque : Inport
  dslip : Inport  Port=2
  enable_tc : Inport  Port=3
  Kp : Inport  Port=4
  Kd : Inport  Port=5
  Add : Sum  Inputs=+-
  Saturation Dynamic : simulink/Discontinuities/Saturation Dynamic  OutMin=[]  OutMax=[]  OutDataTypeStr=Inherit: Same as second input  OutDataType=fixdt(1, 16)  OutScaling=2^-10  DoSatur=off
  min_torque : Constant  Value=0
  traction_controller : Subsystem  TreatAsAtomicUnit=on
  delta_torque : Outport  VectorParamsAs1DForOutWhenUnconnected=off
  wires:
  Kd/1 -> traction_controller/4(Kd)
  enable_tc/1 -> traction_controller/2(enable_tc)
  Kp/1 -> traction_controller/3(Kp)
  traction_controller/1(delta_torque) -> Add/2
  dslip/1 -> traction_controller/1(dslip)
  Saturation Dynamic/1 -> delta_torque/1
  max_torque/1 -> Add/1, Saturation Dynamic/1
  min_torque/1 -> Saturation Dynamic/3
  Add/1 -> Saturation Dynamic/2

== system TorqueVect_HIL_CAN/CarMaker/IPG Vehicle/PowerTrain/PTControl Example/PTControl_TV_MFE25_2022a1/New TC/TC R2/traction_controller ==
  max_torque : Inport
  dslip : Inport  Port=2
  enable_tc : Inport  Port=3
  Kp : Inport  Port=4
  Kd : Inport  Port=5
  Add : Sum  Inputs=+-
  Saturation Dynamic : simulink/Discontinuities/Saturation Dynamic  OutMin=[]  OutMax=[]  OutDataTypeStr=Inherit: Same as second input  OutDataType=fixdt(1, 16)  OutScaling=2^-10  DoSatur=off
  min_torque : Constant  Value=0
  traction_controller : Subsystem  TreatAsAtomicUnit=on
  delta_torque : Outport  VectorParamsAs1DForOutWhenUnconnected=off
  wires:
  Kd/1 -> traction_controller/4(Kd)
  enable_tc/1 -> traction_controller/2(enable_tc)
  Kp/1 -> traction_controller/3(Kp)
  traction_controller/1(delta_torque) -> Add/2
  dslip/1 -> traction_controller/1(dslip)
  Saturation Dynamic/1 -> delta_torque/1
  max_torque/1 -> Add/1, Saturation Dynamic/1
  min_torque/1 -> Saturation Dynamic/3
  Add/1 -> Saturation Dynamic/2

== system TorqueVect_HIL_CAN/CarMaker/IPG Vehicle/PowerTrain/PTControl Example/PTControl_TV_MFE25_2022a1/New TC/TC R3/traction_controller ==
  max_torque : Inport
  dslip : Inport  Port=2
  enable_tc : Inport  Port=3
  Kp : Inport  Port=4
  Kd : Inport  Port=5
  Add : Sum  Inputs=+-
  Saturation Dynamic : simulink/Discontinuities/Saturation Dynamic  OutMin=[]  OutMax=[]  OutDataTypeStr=Inherit: Same as second input  OutDataType=fixdt(1, 16)  OutScaling=2^-10  DoSatur=off
  min_torque : Constant  Value=0
  traction_controller : Subsystem  TreatAsAtomicUnit=on
  delta_torque : Outport  VectorParamsAs1DForOutWhenUnconnected=off
  wires:
  Kd/1 -> traction_controller/4(Kd)
  enable_tc/1 -> traction_controller/2(enable_tc)
  Kp/1 -> traction_controller/3(Kp)
  traction_controller/1(delta_torque) -> Add/2
  dslip/1 -> traction_controller/1(dslip)
  Saturation Dynamic/1 -> delta_torque/1
  max_torque/1 -> Add/1, Saturation Dynamic/1
  min_torque/1 -> Saturation Dynamic/3
  Add/1 -> Saturation Dynamic/2

== system TorqueVect_HIL_CAN/CarMaker/IPG Vehicle/PowerTrain/PTControl Example/PTControl_TV_MFE25_2022a1/New TC/TC R4/traction_controller ==
  max_torque : Inport
  dslip : Inport  Port=2
  enable_tc : Inport  Port=3
  Kp : Inport  Port=4
  Kd : Inport  Port=5
  Add : Sum  Inputs=+-
  Saturation Dynamic : simulink/Discontinuities/Saturation Dynamic  OutMin=[]  OutMax=[]  OutDataTypeStr=Inherit: Same as second input  OutDataType=fixdt(1, 16)  OutScaling=2^-10  DoSatur=off
  min_torque : Constant  Value=0
  traction_controller : Subsystem  TreatAsAtomicUnit=on
  delta_torque : Outport  VectorParamsAs1DForOutWhenUnconnected=off
  wires:
  Kd/1 -> traction_controller/4(Kd)
  enable_tc/1 -> traction_controller/2(enable_tc)
  Kp/1 -> traction_controller/3(Kp)
  traction_controller/1(delta_torque) -> Add/2
  dslip/1 -> traction_controller/1(dslip)
  Saturation Dynamic/1 -> delta_torque/1
  max_torque/1 -> Add/1, Saturation Dynamic/1
  min_torque/1 -> Saturation Dynamic/3
  Add/1 -> Saturation Dynamic/2

== system TorqueVect_HIL_CAN/CarMaker/IPG Vehicle/PowerTrain/PTControl Example/PTControl_TV_MFE3/Full Control Loop/TC 1/Subsystem ==
  velocity : Inport
  pid_kp : Inport  Port=2
  velocity lookup : Inport  Port=3
  pid_ki : Inport  Port=4
  pid_kd : Inport  Port=5
  kd : Lookup_n-D  NumberOfTableDimensions=1  BreakpointsForDimension1Source=Input port  BreakpointsForDimension1=[-5:5]  TableSource=Input port  Table=tanh([-5:5])  InternalRulePriority=Speed  RndMeth=Simplest
      settings: InputPortMap=u0,p221,p5
  ki : Lookup_n-D  NumberOfTableDimensions=1  BreakpointsForDimension1Source=Input port  BreakpointsForDimension1=[-5:5]  TableSource=Input port  Table=tanh([-5:5])  InternalRulePriority=Speed  RndMeth=Simplest
      settings: InputPortMap=u0,p221,p5
  kp : Lookup_n-D  NumberOfTableDimensions=1  BreakpointsForDimension1Source=Input port  BreakpointsForDimension1=[-5:5]  TableSource=Input port  Table=tanh([-5:5])  InternalRulePriority=Speed  RndMeth=Simplest
      settings: InputPortMap=u0,p221,p5
  Out1 : Outport
  Out2 : Outport  Port=2
  Out3 : Outport  Port=3
  wires:
  kp/1 -> Out1/1
  velocity/1 -> kp/1, kd/1, ki/1
  kd/1 -> Out3/1
  ki/1 -> Out2/1
  velocity lookup/1 -> kd/3, ki/3, kp/3
  pid_kp/1 -> kp/2
  pid_ki/1 -> ki/2
  pid_kd/1 -> kd/2

== system TorqueVect_HIL_CAN/CarMaker/IPG Vehicle/PowerTrain/PTControl Example/PTControl_TV_MFE3/Full Control Loop/TC 2/Subsystem ==
  velocity : Inport
  pid_kp : Inport  Port=2
  velocity lookup : Inport  Port=3
  pid_ki : Inport  Port=4
  pid_kd : Inport  Port=5
  kd : Lookup_n-D  NumberOfTableDimensions=1  BreakpointsForDimension1Source=Input port  BreakpointsForDimension1=[-5:5]  TableSource=Input port  Table=tanh([-5:5])  InternalRulePriority=Speed  RndMeth=Simplest
      settings: InputPortMap=u0,p221,p5
  ki : Lookup_n-D  NumberOfTableDimensions=1  BreakpointsForDimension1Source=Input port  BreakpointsForDimension1=[-5:5]  TableSource=Input port  Table=tanh([-5:5])  InternalRulePriority=Speed  RndMeth=Simplest
      settings: InputPortMap=u0,p221,p5
  kp : Lookup_n-D  NumberOfTableDimensions=1  BreakpointsForDimension1Source=Input port  BreakpointsForDimension1=[-5:5]  TableSource=Input port  Table=tanh([-5:5])  InternalRulePriority=Speed  RndMeth=Simplest
      settings: InputPortMap=u0,p221,p5
  Out1 : Outport
  Out2 : Outport  Port=2
  Out3 : Outport  Port=3
  wires:
  kp/1 -> Out1/1
  velocity/1 -> kp/1, kd/1, ki/1
  kd/1 -> Out3/1
  ki/1 -> Out2/1
  velocity lookup/1 -> kd/3, ki/3, kp/3
  pid_kp/1 -> kp/2
  pid_ki/1 -> ki/2
  pid_kd/1 -> kd/2
